simulink subsystem "DetailedBatteryModel"  (R2025b)
settings: Solver=VariableStepAuto  StartTime=0.0  StopTime=10.0  RelTol=1e-3
undefined symbols (not defined in the file): PlntBattBalSwtchThresh, PlntBattBleedRes, PlntBattCondArea, PlntBattNumCellPar, ThrmBatt1, ThrmBatt2, ThrmBatt3, ThrmBatt4
libraries: fl_lib x580, nesl_utility_internal x386, batteryecm_lib x96, simulink x96
(part 2 of 7)

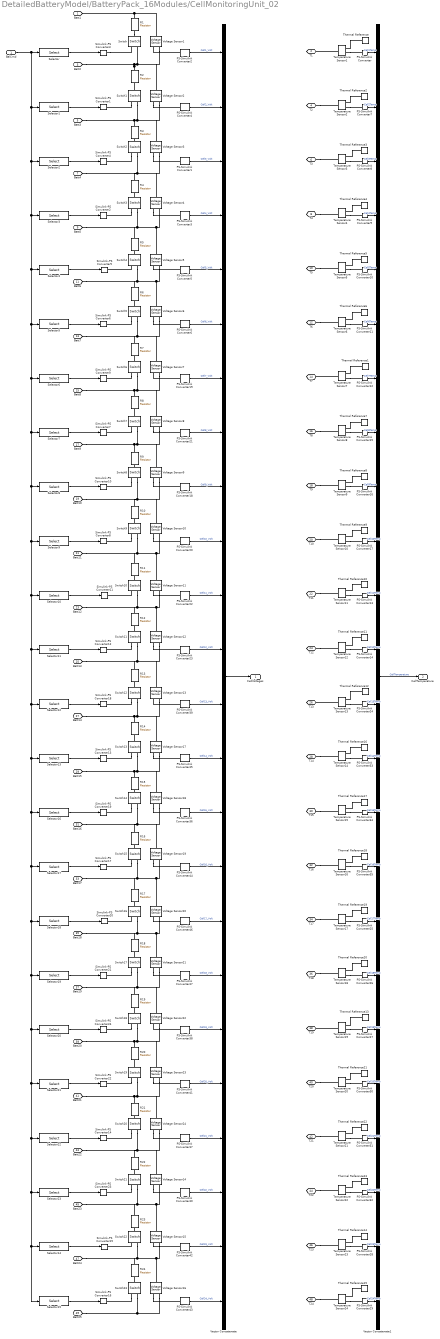
== system DetailedBatteryModel/BatteryPack_16Modules/CellMonitoringUnit_02 ==
  BalCmd : Inport
  PS-Simulink Converter{,7..17,24..35} (24 alike) : nesl_utility_internal/PS-Simulink Converter  PhysicalDomain=network_engine_domain  SubClassName=ps_output  LeftPortType=input  RightPortType=output  PseudoPeriodic=off  Frequencies=[]  VectorFormat=1-D array  Unit=degC  AffineConversion=on
  PS-Simulink Converter{1..6,18..23,36..47} (24 alike) : nesl_utility_internal/PS-Simulink Converter  PhysicalDomain=network_engine_domain  SubClassName=ps_output  LeftPortType=input  RightPortType=output  PseudoPeriodic=off  Frequencies=[]  VectorFormat=1-D array  Unit=V  AffineConversion=off
  R{1..24} (24 alike) : fl_lib/Electrical/Electrical Elements/Resistor  R=PlntBattBleedRes Ohm  i_specify=off  i_priority=None  i=0 A  i_nominal_specify=off  i_nominal_value=1  i_nominal_unit=A  v_specify=off  v_priority=None  v=0 V  v_nominal_specify=off  v_nominal_value=1  v_nominal_unit=V
      R1 settings: LogSimulationData=on
      R13 settings: LogSimulationData=on
      R19 settings: LogSimulationData=on
      R7 settings: LogSimulationData=on
  Selector : Selector  IndexOptions=Index vector (dialog)  Indices=1  OutputSizes=1
  Selector1 : Selector  IndexOptions=Index vector (dialog)  Indices=2  OutputSizes=1
  Selector10 : Selector  IndexOptions=Index vector (dialog)  Indices=11  OutputSizes=1
  Selector11 : Selector  IndexOptions=Index vector (dialog)  Indices=12  OutputSizes=1
  Selector12 : Selector  IndexOptions=Index vector (dialog)  Indices=13  OutputSizes=1
  Selector13 : Selector  IndexOptions=Index vector (dialog)  Indices=14  OutputSizes=1
  Selector14 : Selector  IndexOptions=Index vector (dialog)  Indices=23  OutputSizes=1
  Selector15 : Selector  IndexOptions=Index vector (dialog)  Indices=24  OutputSizes=1
  Selector16 : Selector  IndexOptions=Index vector (dialog)  Indices=15  OutputSizes=1
  Selector17 : Selector  IndexOptions=Index vector (dialog)  Indices=16  OutputSizes=1
  Selector18 : Selector  IndexOptions=Index vector (dialog)  Indices=17  OutputSizes=1
  Selector19 : Selector  IndexOptions=Index vector (dialog)  Indices=18  OutputSizes=1
  Selector2 : Selector  IndexOptions=Index vector (dialog)  Indices=3  OutputSizes=1
  Selector20 : Selector  IndexOptions=Index vector (dialog)  Indices=19  OutputSizes=1
  Selector21 : Selector  IndexOptions=Index vector (dialog)  Indices=20  OutputSizes=1
  Selector22 : Selector  IndexOptions=Index vector (dialog)  Indices=21  OutputSizes=1
  Selector23 : Selector  IndexOptions=Index vector (dialog)  Indices=22  OutputSizes=1
  Selector3 : Selector  IndexOptions=Index vector (dialog)  Indices=4  OutputSizes=1
  Selector4 : Selector  IndexOptions=Index vector (dialog)  Indices=5  OutputSizes=1
  Selector5 : Selector  IndexOptions=Index vector (dialog)  Indices=6  OutputSizes=1
  Selector6 : Selector  IndexOptions=Index vector (dialog)  Indices=7  OutputSizes=1
  Selector7 : Selector  IndexOptions=Index vector (dialog)  Indices=8  OutputSizes=1
  Selector8 : Selector  IndexOptions=Index vector (dialog)  Indices=9  OutputSizes=1
  Selector9 : Selector  IndexOptions=Index vector (dialog)  Indices=10  OutputSizes=1
  Simulink-PS Converter{1..24} (24 alike) : nesl_utility_internal/Simulink-PS Converter  PhysicalDomain=network_engine_domain  SubClassName=ps_input  LeftPortType=input  RightPortType=output  PseudoPeriodic=off  Frequencies=[]  NoiseDistribution=none  NoiseParameters=[]  Unit=1  AffineConversion=off  FilteringAndDerivatives=zero  SimscapeFilterOrder=1  InputFilterTimeConstant=0.001  UdotUserProvided=1
  Switch{,1..23} (24 alike) : fl_lib/Electrical/Electrical Elements/Switch  R_closed=PlntBattBalSwtchClsdRes Ohm  G_open=PlntBattBalSwtchOpenCond 1/Ohm  Threshold=PlntBattBalSwtchThresh  i_specify=off  i_priority=None  i=0 A  i_nominal_specify=off  i_nominal_value=1  i_nominal_unit=A  v_specify=off  v_priority=None  v=0 V  v_nominal_specify=off  v_nominal_value=1  v_nominal_unit=V
  Temperature Sensor{1..24} (24 alike) : fl_lib/Thermal/Thermal Sensors/Temperature Sensor  temperature_measure=foundation.enum.MeasurementReference.difference
  Thermal Reference{,1..23} (24 alike) : fl_lib/Thermal/Thermal Elements/Thermal Reference
  Vector Concatenate : Concatenate  NumInputs=24
  Vector Concatenate1 : Concatenate  NumInputs=24
  Voltage Sensor{1..24} (24 alike) : fl_lib/Electrical/Electrical Sensors/Voltage Sensor
  Batt1 : PMIOPort  Side=Left
  T1 : PMIOPort  Port=2  Side=Left
  Batt2 : PMIOPort  Port=3  Side=Left
  T2 : PMIOPort  Port=4  Side=Left
  Batt3 : PMIOPort  Port=5  Side=Left
  T3 : PMIOPort  Port=6  Side=Left
  Batt4 : PMIOPort  Port=7  Side=Left
  T4 : PMIOPort  Port=8  Side=Left
  Batt5 : PMIOPort  Port=9  Side=Left
  T5 : PMIOPort  Port=10  Side=Left
  Batt6 : PMIOPort  Port=11  Side=Left
  T6 : PMIOPort  Port=12  Side=Left
  Batt7 : PMIOPort  Port=13  Side=Left
  T7 : PMIOPort  Port=14  Side=Left
  Batt8 : PMIOPort  Port=15  Side=Left
  T8 : PMIOPort  Port=16  Side=Left
  Batt9 : PMIOPort  Port=17  Side=Left
  T9 : PMIOPort  Port=18  Side=Left
  Batt10 : PMIOPort  Port=19  Side=Left
  T10 : PMIOPort  Port=20  Side=Left
  Batt11 : PMIOPort  Port=21  Side=Left
  T11 : PMIOPort  Port=22  Side=Left
  Batt12 : PMIOPort  Port=23  Side=Left
  T12 : PMIOPort  Port=24  Side=Left
  Batt13 : PMIOPort  Port=25  Side=Left
  T13 : PMIOPort  Port=26  Side=Left
  Batt14 : PMIOPort  Port=27  Side=Left
  T14 : PMIOPort  Port=28  Side=Left
  Batt15 : PMIOPort  Port=29  Side=Left
  T15 : PMIOPort  Port=30  Side=Left
  Batt16 : PMIOPort  Port=31  Side=Left
  T16 : PMIOPort  Port=32  Side=Left
  Batt17 : PMIOPort  Port=33  Side=Left
  T17 : PMIOPort  Port=34  Side=Left
  Batt18 : PMIOPort  Port=35  Side=Left
  T18 : PMIOPort  Port=36  Side=Left
  Batt19 : PMIOPort  Port=37  Side=Left
  T19 : PMIOPort  Port=38  Side=Left
  Batt20 : PMIOPort  Port=39  Side=Left
  T20 : PMIOPort  Port=40  Side=Left
  Batt21 : PMIOPort  Port=41  Side=Left
  T21 : PMIOPort  Port=42  Side=Left
  Batt22 : PMIOPort  Port=43  Side=Left
  T22 : PMIOPort  Port=44  Side=Left
  Batt23 : PMIOPort  Port=45  Side=Left
  T23 : PMIOPort  Port=46  Side=Left
  Batt24 : PMIOPort  Port=47  Side=Left
  T24 : PMIOPort  Port=48  Side=Left
  Batt25 : PMIOPort  Port=49  Side=Left
  CellVoltages : Outport  VectorParamsAs1DForOutWhenUnconnected=off
  CellTemperature : Outport  Port=2  VectorParamsAs1DForOutWhenUnconnected=off
  wires:
  PS-Simulink Converter11/1 -> Vector Concatenate1/6  "Cell6Temp"
  PS-Simulink Converter10/1 -> Vector Concatenate1/5  "Cell5Temp"
  PS-Simulink Converter8/1 -> Vector Concatenate1/3  "Cell3Temp"
  PS-Simulink Converter7/1 -> Vector Concatenate1/2  "Cell2Temp"
  PS-Simulink Converter9/1 -> Vector Concatenate1/4  "Cell4Temp"
  PS-Simulink Converter/1 -> Vector Concatenate1/1  "Cell1Temp"
  Vector Concatenate1/1 -> CellTemperature/1  "CellTemperature"
  PS-Simulink Converter6/1 -> Vector Concatenate/6  "Cell6_Volt"
  PS-Simulink Converter5/1 -> Vector Concatenate/5  "Cell5_Volt"
  PS-Simulink Converter3/1 -> Vector Concatenate/4  "Cell4_Volt"
  PS-Simulink Converter1/1 -> Vector Concatenate/3  "Cell3_Volt"
  PS-Simulink Converter4/1 -> Vector Concatenate/2  "Cell2_Volt"
  PS-Simulink Converter2/1 -> Vector Concatenate/1  "Cell1_Volt"
  Selector5/1 -> Simulink-PS Converter6/1
  Selector4/1 -> Simulink-PS Converter5/1
  Selector3/1 -> Simulink-PS Converter2/1
  Selector/1 -> Simulink-PS Converter3/1
  Selector1/1 -> Simulink-PS Converter1/1
  Selector2/1 -> Simulink-PS Converter4/1
  Vector Concatenate/1 -> CellVoltages/1
  PS-Simulink Converter12/1 -> Vector Concatenate1/7  "Cell7Temp"
  PS-Simulink Converter15/1 -> Vector Concatenate1/8  "Cell8Temp"
  PS-Simulink Converter13/1 -> Vector Concatenate1/11  "Cell11Temp"
  PS-Simulink Converter17/1 -> Vector Concatenate1/10  "Cell10Temp"
  PS-Simulink Converter16/1 -> Vector Concatenate1/9  "Cell9Temp"
  PS-Simulink Converter14/1 -> Vector Concatenate1/12  "Cell12Temp"
  PS-Simulink Converter20/1 -> Vector Concatenate/10  "Cell10_Volt"
  Selector9/1 -> Simulink-PS Converter8/1
  Selector11/1 -> Simulink-PS Converter12/1
  Selector6/1 -> Simulink-PS Converter9/1
  PS-Simulink Converter18/1 -> Vector Concatenate/9  "Cell9_Volt"
  Selector8/1 -> Simulink-PS Converter10/1
  Selector7/1 -> Simulink-PS Converter7/1
  PS-Simulink Converter22/1 -> Vector Concatenate/11  "Cell11_Volt"
  PS-Simulink Converter23/1 -> Vector Concatenate/12  "Cell12_Volt"
  PS-Simulink Converter19/1 -> Vector Concatenate/7  "Cell7_Volt"
  PS-Simulink Converter21/1 -> Vector Concatenate/8  "Cell8_Volt"
  Selector10/1 -> Simulink-PS Converter11/1
  PS-Simulink Converter24/1 -> Vector Concatenate1/13  "Cell13Temp"
  PS-Simulink Converter33/1 -> Vector Concatenate1/14  "Cell14Temp"
  PS-Simulink Converter25/1 -> Vector Concatenate1/17  "Cell17Temp"
  PS-Simulink Converter30/1 -> Vector Concatenate1/20  "Cell20Temp"
  PS-Simulink Converter31/1 -> Vector Concatenate1/21  "Cell21Temp"
  PS-Simulink Converter28/1 -> Vector Concatenate1/23  "Cell23Temp"
  PS-Simulink Converter29/1 -> Vector Concatenate1/24  "Cell24Temp"
  PS-Simulink Converter27/1 -> Vector Concatenate1/19  "Cell19Temp"
  PS-Simulink Converter26/1 -> Vector Concatenate1/18  "Cell18Temp"
  PS-Simulink Converter34/1 -> Vector Concatenate1/15  "Cell15Temp"
  PS-Simulink Converter35/1 -> Vector Concatenate1/16  "Cell16Temp"
  PS-Simulink Converter32/1 -> Vector Concatenate1/22  "Cell22Temp"
  PS-Simulink Converter44/1 -> Vector Concatenate/16  "Cell16_Volt"
  Selector17/1 -> Simulink-PS Converter17/1
  Selector19/1 -> Simulink-PS Converter21/1
  Selector12/1 -> Simulink-PS Converter18/1
  PS-Simulink Converter36/1 -> Vector Concatenate/15  "Cell15_Volt"
  Selector13/1 -> Simulink-PS Converter13/1
  BalCmd/1 -> Selector/1, Selector1/1, Selector2/1, Selector4/1, Selector6/1, Selector7/1, Selector8/1, Selector10/1, Selector13/1, Selector16/1, Selector18/1, Selector20/1, Selector21/1, Selector22/1, Selector14/1, Selector15/1, Selector23/1, Selector19/1, Selector17/1, Selector12/1, Selector11/1, Selector9/1, Selector5/1, Selector3/1
  PS-Simulink Converter37/1 -> Vector Concatenate/21  "Cell21_Volt"
  PS-Simulink Converter38/1 -> Vector Concatenate/19  "Cell19_Volt"
  PS-Simulink Converter41/1 -> Vector Concatenate/20  "Cell20_Volt"
  PS-Simulink Converter43/1 -> Vector Concatenate/24  "Cell24_Volt"
  Selector15/1 -> Simulink-PS Converter16/1
  Selector20/1 -> Simulink-PS Converter24/1
  Selector22/1 -> Simulink-PS Converter14/1
  Selector14/1 -> Simulink-PS Converter15/1
  Selector21/1 -> Simulink-PS Converter22/1
  PS-Simulink Converter42/1 -> Vector Concatenate/23  "Cell23_Volt"
  Selector16/1 -> Simulink-PS Converter19/1
  PS-Simulink Converter46/1 -> Vector Concatenate/17  "Cell17_Volt"
  PS-Simulink Converter40/1 -> Vector Concatenate/22  "Cell22_Volt"
  PS-Simulink Converter47/1 -> Vector Concatenate/18  "Cell18_Volt"
  Selector23/1 -> Simulink-PS Converter23/1
  PS-Simulink Converter45/1 -> Vector Concatenate/14  "Cell14_Volt"
  Selector18/1 -> Simulink-PS Converter20/1
  PS-Simulink Converter39/1 -> Vector Concatenate/13  "Cell13_Volt"
  connections:
  Thermal Reference/LConn1 -- Temperature Sensor1/RConn1
  T6/RConn1 -- Temperature Sensor6/LConn1
  T5/RConn1 -- Temperature Sensor5/LConn1
  T4/RConn1 -- Temperature Sensor4/LConn1
  T3/RConn1 -- Temperature Sensor3/LConn1
  T2/RConn1 -- Temperature Sensor2/LConn1
  Temperature Sensor1/LConn1 -- T1/RConn1
  Thermal Reference5/LConn1 -- Temperature Sensor5/RConn1
  Thermal Reference2/LConn1 -- Temperature Sensor2/RConn1
  Thermal Reference6/LConn1 -- Temperature Sensor6/RConn1
  Temperature Sensor2/RConn2 -- PS-Simulink Converter7/LConn1
  Thermal Reference4/LConn1 -- Temperature Sensor4/RConn1
  Temperature Sensor5/RConn2 -- PS-Simulink Converter10/LConn1
  Thermal Reference3/LConn1 -- Temperature Sensor3/RConn1
  Temperature Sensor4/RConn2 -- PS-Simulink Converter9/LConn1
  Temperature Sensor6/RConn2 -- PS-Simulink Converter11/LConn1
  Temperature Sensor1/RConn2 -- PS-Simulink Converter/LConn1
  Temperature Sensor3/RConn2 -- PS-Simulink Converter8/LConn1
  Voltage Sensor6/RConn1 -- PS-Simulink Converter6/LConn1
  Voltage Sensor5/RConn1 -- PS-Simulink Converter5/LConn1
  Voltage Sensor4/RConn1 -- PS-Simulink Converter3/LConn1
  Switch5/LConn1 -- R6/RConn1
  Switch5/RConn1 -- Simulink-PS Converter6/RConn1
  Switch5/RConn2 -- R7/LConn1 -- Batt7/RConn1 -- Voltage Sensor6/RConn2 -- Voltage Sensor7/LConn1
  Switch4/LConn1 -- R5/RConn1
  Switch4/RConn1 -- Simulink-PS Converter5/RConn1
  Switch4/RConn2 -- Voltage Sensor5/RConn2 -- Voltage Sensor6/LConn1 -- R6/LConn1 -- Batt6/RConn1
  Switch3/RConn1 -- Simulink-PS Converter2/RConn1
  Switch3/LConn1 -- R4/RConn1
  Switch3/RConn2 -- Batt5/RConn1 -- R5/LConn1 -- Voltage Sensor5/LConn1 -- Voltage Sensor4/RConn2
  Switch1/RConn2 -- R3/LConn1 -- Batt3/RConn1 -- Voltage Sensor2/RConn2 -- Voltage Sensor3/LConn1
  R2/LConn1 -- Switch/RConn2 -- Voltage Sensor1/RConn2 -- Voltage Sensor2/LConn1 -- Batt2/RConn1
  R1/RConn1 -- Switch/LConn1
  Switch2/LConn1 -- R3/RConn1
  R1/LConn1 -- Voltage Sensor1/LConn1 -- Batt1/RConn1
  PS-Simulink Converter2/LConn1 -- Voltage Sensor1/RConn1
  Voltage Sensor2/RConn1 -- PS-Simulink Converter4/LConn1
  Switch1/LConn1 -- R2/RConn1
  Simulink-PS Converter3/RConn1 -- Switch/RConn1
  Switch1/RConn1 -- Simulink-PS Converter1/RConn1
  Switch2/RConn1 -- Simulink-PS Converter4/RConn1
  Voltage Sensor3/RConn1 -- PS-Simulink Converter1/LConn1
  Switch2/RConn2 -- R4/LConn1 -- Batt4/RConn1 -- Voltage Sensor3/RConn2 -- Voltage Sensor4/LConn1
  Temperature Sensor8/RConn2 -- PS-Simulink Converter15/LConn1
  Temperature Sensor11/RConn2 -- PS-Simulink Converter13/LConn1
  Thermal Reference9/LConn1 -- Temperature Sensor10/RConn1
  Temperature Sensor9/RConn2 -- PS-Simulink Converter16/LConn1
  Temperature Sensor10/RConn2 -- PS-Simulink Converter17/LConn1
  Thermal Reference11/LConn1 -- Temperature Sensor12/RConn1
  T10/RConn1 -- Temperature Sensor10/LConn1
  Thermal Reference10/LConn1 -- Temperature Sensor11/RConn1
  Temperature Sensor12/RConn2 -- PS-Simulink Converter14/LConn1
  Thermal Reference1/LConn1 -- Temperature Sensor7/RConn1
  T8/RConn1 -- Temperature Sensor8/LConn1
  Temperature Sensor7/LConn1 -- T7/RConn1
  T9/RConn1 -- Temperature Sensor9/LConn1
  T11/RConn1 -- Temperature Sensor11/LConn1
  Thermal Reference7/LConn1 -- Temperature Sensor8/RConn1
  T12/RConn1 -- Temperature Sensor12/LConn1
  Temperature Sensor7/RConn2 -- PS-Simulink Converter12/LConn1
  Thermal Reference8/LConn1 -- Temperature Sensor9/RConn1
  Switch8/RConn2 -- Voltage Sensor9/RConn2 -- Voltage Sensor10/LConn1 -- R10/LConn1 -- Batt10/RConn1
  Switch6/RConn2 -- R8/LConn1 -- Batt8/RConn1 -- Voltage Sensor7/RConn2 -- Voltage Sensor8/LConn1
  Switch10/RConn2 -- R12/LConn1 -- Batt12/RConn1 -- Voltage Sensor12/LConn1 -- Voltage Sensor11/RConn2
  Switch9/RConn2 -- Voltage Sensor10/RConn2 -- Voltage Sensor11/LConn1 -- R11/LConn1 -- Batt11/RConn1
  Switch7/RConn2 -- Voltage Sensor9/LConn1 -- Voltage Sensor8/RConn2 -- Batt9/RConn1 -- R9/LConn1
  Switch11/RConn2 -- R13/LConn1 -- Batt13/RConn1 -- Voltage Sensor12/RConn2 -- Voltage Sensor13/LConn1
  Switch9/LConn1 -- R10/RConn1
  Switch7/RConn1 -- Simulink-PS Converter7/RConn1
  Switch6/LConn1 -- R7/RConn1
  Voltage Sensor12/RConn1 -- PS-Simulink Converter23/LConn1
  Voltage Sensor10/RConn1 -- PS-Simulink Converter20/LConn1
  Switch7/LConn1 -- R8/RConn1
  Voltage Sensor8/RConn1 -- PS-Simulink Converter21/LConn1
  Voltage Sensor9/RConn1 -- PS-Simulink Converter18/LConn1
  Switch6/RConn1 -- Simulink-PS Converter9/RConn1
  PS-Simulink Converter19/LConn1 -- Voltage Sensor7/RConn1
  Switch8/LConn1 -- R9/RConn1
  Voltage Sensor11/RConn1 -- PS-Simulink Converter22/LConn1
  Switch9/RConn1 -- Simulink-PS Converter8/RConn1
  Switch10/RConn1 -- Simulink-PS Converter11/RConn1
  Switch10/LConn1 -- R11/RConn1
  Switch11/RConn1 -- Simulink-PS Converter12/RConn1
  Switch11/LConn1 -- R12/RConn1
  Switch8/RConn1 -- Simulink-PS Converter10/RConn1
  Thermal Reference20/LConn1 -- Temperature Sensor18/RConn1
  T16/RConn1 -- Temperature Sensor16/LConn1
  Thermal Reference18/LConn1 -- Temperature Sensor16/RConn1
  Thermal Reference19/LConn1 -- Temperature Sensor17/RConn1
  T17/RConn1 -- Temperature Sensor17/LConn1
  Temperature Sensor13/LConn1 -- T13/RConn1
  Temperature Sensor17/RConn2 -- PS-Simulink Converter25/LConn1
  Temperature Sensor16/RConn2 -- PS-Simulink Converter35/LConn1
  Thermal Reference16/LConn1 -- Temperature Sensor14/RConn1
  T20/RConn1 -- Temperature Sensor20/LConn1
  Temperature Sensor15/RConn2 -- PS-Simulink Converter34/LConn1
  Thermal Reference17/LConn1 -- Temperature Sensor15/RConn1
  Temperature Sensor21/RConn2 -- PS-Simulink Converter31/LConn1
  Thermal Reference13/LConn1 -- Temperature Sensor19/RConn1
  Thermal Reference14/LConn1 -- Temperature Sensor23/RConn1
  Thermal Reference15/LConn1 -- Temperature Sensor24/RConn1
  Thermal Reference12/LConn1 -- Temperature Sensor13/RConn1
  Temperature Sensor18/RConn2 -- PS-Simulink Converter26/LConn1
  T14/RConn1 -- Temperature Sensor14/LConn1
  T22/RConn1 -- Temperature Sensor22/LConn1
  Thermal Reference23/LConn1 -- Temperature Sensor22/RConn1
  Temperature Sensor13/RConn2 -- PS-Simulink Converter24/LConn1
  Temperature Sensor24/RConn2 -- PS-Simulink Converter29/LConn1
  Thermal Reference22/LConn1 -- Temperature Sensor21/RConn1
  T21/RConn1 -- Temperature Sensor21/LConn1
  T18/RConn1 -- Temperature Sensor18/LConn1
  T15/RConn1 -- Temperature Sensor15/LConn1
  T23/RConn1 -- Temperature Sensor23/LConn1
  T24/RConn1 -- Temperature Sensor24/LConn1
  Temperature Sensor19/LConn1 -- T19/RConn1
  Temperature Sensor23/RConn2 -- PS-Simulink Converter28/LConn1
  Temperature Sensor19/RConn2 -- PS-Simulink Converter27/LConn1
  Temperature Sensor14/RConn2 -- PS-Simulink Converter33/LConn1
  Thermal Reference21/LConn1 -- Temperature Sensor20/RConn1
  Temperature Sensor20/RConn2 -- PS-Simulink Converter30/LConn1
  Temperature Sensor22/RConn2 -- PS-Simulink Converter32/LConn1
  Switch20/RConn2 -- Voltage Sensor24/RConn2 -- Voltage Sensor14/LConn1 -- R22/LConn1 -- Batt22/RConn1
  Switch16/RConn2 -- R18/LConn1 -- Batt18/RConn1 -- Voltage Sensor21/LConn1 -- Voltage Sensor20/RConn2
  Switch14/RConn2 -- R16/LConn1 -- Batt16/RConn1 -- Voltage Sensor19/LConn1 -- Voltage Sensor18/RConn2
  Switch22/RConn2 -- R24/LConn1 -- Batt24/RConn1 -- Voltage Sensor16/LConn1 -- Voltage Sensor15/RConn2
  Switch19/RConn2 -- Voltage Sensor24/LConn1 -- Voltage Sensor23/RConn2 -- Batt21/RConn1 -- R21/LConn1
  Switch21/RConn2 -- Voltage Sensor14/RConn2 -- Voltage Sensor15/LConn1 -- Batt23/RConn1 -- R23/LConn1
  Switch12/RConn2 -- R14/LConn1 -- Batt14/RConn1 -- Voltage Sensor13/RConn2 -- Voltage Sensor17/LConn1
  Switch15/RConn2 -- Voltage Sensor19/RConn2 -- Voltage Sensor20/LConn1 -- R17/LConn1 -- Batt17/RConn1
  Switch13/RConn2 -- R15/LConn1 -- Batt15/RConn1 -- Voltage Sensor18/LConn1 -- Voltage Sensor17/RConn2
  Switch17/RConn2 -- R19/LConn1 -- Batt19/RConn1 -- Voltage Sensor21/RConn2 -- Voltage Sensor22/LConn1
  Switch18/RConn2 -- Voltage Sensor22/RConn2 -- Voltage Sensor23/LConn1 -- Batt20/RConn1 -- R20/LConn1
  Switch23/RConn2 -- Batt25/RConn1 -- Voltage Sensor16/RConn2
  Switch14/RConn1 -- Simulink-PS Converter19/RConn1
  Switch22/RConn1 -- Simulink-PS Converter15/RConn1
  Voltage Sensor21/RConn1 -- PS-Simulink Converter47/LConn1
  Switch13/LConn1 -- R14/RConn1
  PS-Simulink Converter39/LConn1 -- Voltage Sensor13/RConn1
  Voltage Sensor19/RConn1 -- PS-Simulink Converter44/LConn1
  Switch21/RConn1 -- Simulink-PS Converter23/RConn1
  Voltage Sensor23/RConn1 -- PS-Simulink Converter41/LConn1
  Voltage Sensor18/RConn1 -- PS-Simulink Converter36/LConn1
  Voltage Sensor17/RConn1 -- PS-Simulink Converter45/LConn1
  Switch23/LConn1 -- R24/RConn1
  Switch12/LConn1 -- R13/RConn1
  PS-Simulink Converter38/LConn1 -- Voltage Sensor22/RConn1
  Switch18/RConn1 -- Simulink-PS Converter24/RConn1
  Switch12/RConn1 -- Simulink-PS Converter18/RConn1
  Switch13/RConn1 -- Simulink-PS Converter13/RConn1
  Switch15/LConn1 -- R16/RConn1
  Switch20/LConn1 -- R21/RConn1
  Switch14/LConn1 -- R15/RConn1
  Voltage Sensor14/RConn1 -- PS-Simulink Converter40/LConn1
  Voltage Sensor20/RConn1 -- PS-Simulink Converter46/LConn1
  Voltage Sensor16/RConn1 -- PS-Simulink Converter43/LConn1
  Switch18/LConn1 -- R19/RConn1
  Switch21/LConn1 -- R22/RConn1
  Switch17/LConn1 -- R18/RConn1
  Switch16/RConn1 -- Simulink-PS Converter20/RConn1
  Switch19/RConn1 -- Simulink-PS Converter22/RConn1
  Switch16/LConn1 -- R17/RConn1
  Voltage Sensor15/RConn1 -- PS-Simulink Converter42/LConn1
  Switch17/RConn1 -- Simulink-PS Converter21/RConn1
  Switch23/RConn1 -- Simulink-PS Converter16/RConn1
  Switch20/RConn1 -- Simulink-PS Converter14/RConn1
  Switch22/LConn1 -- R23/RConn1
  Switch19/LConn1 -- R20/RConn1
  Switch15/RConn1 -- Simulink-PS Converter17/RConn1
  Voltage Sensor24/RConn1 -- PS-Simulink Converter37/LConn1

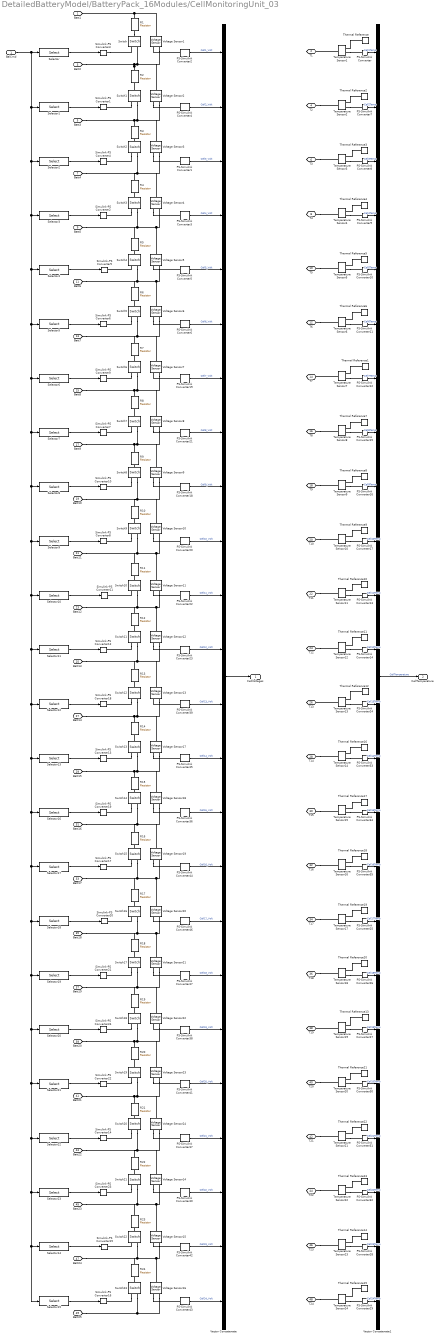
== system DetailedBatteryModel/BatteryPack_16Modules/CellMonitoringUnit_03 ==
  BalCmd : Inport
  PS-Simulink Converter{,7..17,24..35} (24 alike) : nesl_utility_internal/PS-Simulink Converter  PhysicalDomain=network_engine_domain  SubClassName=ps_output  LeftPortType=input  RightPortType=output  PseudoPeriodic=off  Frequencies=[]  VectorFormat=1-D array  Unit=degC  AffineConversion=on
  PS-Simulink Converter{1..6,18..23,36..47} (24 alike) : nesl_utility_internal/PS-Simulink Converter  PhysicalDomain=network_engine_domain  SubClassName=ps_output  LeftPortType=input  RightPortType=output  PseudoPeriodic=off  Frequencies=[]  VectorFormat=1-D array  Unit=V  AffineConversion=off
  R{1..24} (24 alike) : fl_lib/Electrical/Electrical Elements/Resistor  R=PlntBattBleedRes Ohm  i_specify=off  i_priority=None  i=0 A  i_nominal_specify=off  i_nominal_value=1  i_nominal_unit=A  v_specify=off  v_priority=None  v=0 V  v_nominal_specify=off  v_nominal_value=1  v_nominal_unit=V
      R1 settings: LogSimulationData=on
      R13 settings: LogSimulationData=on
      R19 settings: LogSimulationData=on
      R7 settings: LogSimulationData=on
  Selector : Selector  IndexOptions=Index vector (dialog)  Indices=1  OutputSizes=1
  Selector1 : Selector  IndexOptions=Index vector (dialog)  Indices=2  OutputSizes=1
  Selector10 : Selector  IndexOptions=Index vector (dialog)  Indices=11  OutputSizes=1
  Selector11 : Selector  IndexOptions=Index vector (dialog)  Indices=12  OutputSizes=1
  Selector12 : Selector  IndexOptions=Index vector (dialog)  Indices=13  OutputSizes=1
  Selector13 : Selector  IndexOptions=Index vector (dialog)  Indices=14  OutputSizes=1
  Selector14 : Selector  IndexOptions=Index vector (dialog)  Indices=23  OutputSizes=1
  Selector15 : Selector  IndexOptions=Index vector (dialog)  Indices=24  OutputSizes=1
  Selector16 : Selector  IndexOptions=Index vector (dialog)  Indices=15  OutputSizes=1
  Selector17 : Selector  IndexOptions=Index vector (dialog)  Indices=16  OutputSizes=1
  Selector18 : Selector  IndexOptions=Index vector (dialog)  Indices=17  OutputSizes=1
  Selector19 : Selector  IndexOptions=Index vector (dialog)  Indices=18  OutputSizes=1
  Selector2 : Selector  IndexOptions=Index vector (dialog)  Indices=3  OutputSizes=1
  Selector20 : Selector  IndexOptions=Index vector (dialog)  Indices=19  OutputSizes=1
  Selector21 : Selector  IndexOptions=Index vector (dialog)  Indices=20  OutputSizes=1
  Selector22 : Selector  IndexOptions=Index vector (dialog)  Indices=21  OutputSizes=1
  Selector23 : Selector  IndexOptions=Index vector (dialog)  Indices=22  OutputSizes=1
  Selector3 : Selector  IndexOptions=Index vector (dialog)  Indices=4  OutputSizes=1
  Selector4 : Selector  IndexOptions=Index vector (dialog)  Indices=5  OutputSizes=1
  Selector5 : Selector  IndexOptions=Index vector (dialog)  Indices=6  OutputSizes=1
  Selector6 : Selector  IndexOptions=Index vector (dialog)  Indices=7  OutputSizes=1
  Selector7 : Selector  IndexOptions=Index vector (dialog)  Indices=8  OutputSizes=1
  Selector8 : Selector  IndexOptions=Index vector (dialog)  Indices=9  OutputSizes=1
  Selector9 : Selector  IndexOptions=Index vector (dialog)  Indices=10  OutputSizes=1
  Simulink-PS Converter{1..24} (24 alike) : nesl_utility_internal/Simulink-PS Converter  PhysicalDomain=network_engine_domain  SubClassName=ps_input  LeftPortType=input  RightPortType=output  PseudoPeriodic=off  Frequencies=[]  NoiseDistribution=none  NoiseParameters=[]  Unit=1  AffineConversion=off  FilteringAndDerivatives=zero  SimscapeFilterOrder=1  InputFilterTimeConstant=0.001  UdotUserProvided=1
  Switch{,1..23} (24 alike) : fl_lib/Electrical/Electrical Elements/Switch  R_closed=PlntBattBalSwtchClsdRes Ohm  G_open=PlntBattBalSwtchOpenCond 1/Ohm  Threshold=PlntBattBalSwtchThresh  i_specify=off  i_priority=None  i=0 A  i_nominal_specify=off  i_nominal_value=1  i_nominal_unit=A  v_specify=off  v_priority=None  v=0 V  v_nominal_specify=off  v_nominal_value=1  v_nominal_unit=V
  Temperature Sensor{1..24} (24 alike) : fl_lib/Thermal/Thermal Sensors/Temperature Sensor  temperature_measure=foundation.enum.MeasurementReference.difference
  Thermal Reference{,1..23} (24 alike) : fl_lib/Thermal/Thermal Elements/Thermal Reference
  Vector Concatenate : Concatenate  NumInputs=24
  Vector Concatenate1 : Concatenate  NumInputs=24
  Voltage Sensor{1..24} (24 alike) : fl_lib/Electrical/Electrical Sensors/Voltage Sensor
  Batt1 : PMIOPort  Side=Left
  T1 : PMIOPort  Port=2  Side=Left
  Batt2 : PMIOPort  Port=3  Side=Left
  T2 : PMIOPort  Port=4  Side=Left
  Batt3 : PMIOPort  Port=5  Side=Left
  T3 : PMIOPort  Port=6  Side=Left
  Batt4 : PMIOPort  Port=7  Side=Left
  T4 : PMIOPort  Port=8  Side=Left
  Batt5 : PMIOPort  Port=9  Side=Left
  T5 : PMIOPort  Port=10  Side=Left
  Batt6 : PMIOPort  Port=11  Side=Left
  T6 : PMIOPort  Port=12  Side=Left
  Batt7 : PMIOPort  Port=13  Side=Left
  T7 : PMIOPort  Port=14  Side=Left
  Batt8 : PMIOPort  Port=15  Side=Left
  T8 : PMIOPort  Port=16  Side=Left
  Batt9 : PMIOPort  Port=17  Side=Left
  T9 : PMIOPort  Port=18  Side=Left
  Batt10 : PMIOPort  Port=19  Side=Left
  T10 : PMIOPort  Port=20  Side=Left
  Batt11 : PMIOPort  Port=21  Side=Left
  T11 : PMIOPort  Port=22  Side=Left
  Batt12 : PMIOPort  Port=23  Side=Left
  T12 : PMIOPort  Port=24  Side=Left
  Batt13 : PMIOPort  Port=25  Side=Left
  T13 : PMIOPort  Port=26  Side=Left
  Batt14 : PMIOPort  Port=27  Side=Left
  T14 : PMIOPort  Port=28  Side=Left
  Batt15 : PMIOPort  Port=29  Side=Left
  T15 : PMIOPort  Port=30  Side=Left
  Batt16 : PMIOPort  Port=31  Side=Left
  T16 : PMIOPort  Port=32  Side=Left
  Batt17 : PMIOPort  Port=33  Side=Left
  T17 : PMIOPort  Port=34  Side=Left
  Batt18 : PMIOPort  Port=35  Side=Left
  T18 : PMIOPort  Port=36  Side=Left
  Batt19 : PMIOPort  Port=37  Side=Left
  T19 : PMIOPort  Port=38  Side=Left
  Batt20 : PMIOPort  Port=39  Side=Left
  T20 : PMIOPort  Port=40  Side=Left
  Batt21 : PMIOPort  Port=41  Side=Left
  T21 : PMIOPort  Port=42  Side=Left
  Batt22 : PMIOPort  Port=43  Side=Left
  T22 : PMIOPort  Port=44  Side=Left
  Batt23 : PMIOPort  Port=45  Side=Left
  T23 : PMIOPort  Port=46  Side=Left
  Batt24 : PMIOPort  Port=47  Side=Left
  T24 : PMIOPort  Port=48  Side=Left
  Batt25 : PMIOPort  Port=49  Side=Left
  CellVoltages : Outport  VectorParamsAs1DForOutWhenUnconnected=off
  CellTemperature : Outport  Port=2  VectorParamsAs1DForOutWhenUnconnected=off
  wires:
  PS-Simulink Converter11/1 -> Vector Concatenate1/6  "Cell6Temp"
  PS-Simulink Converter10/1 -> Vector Concatenate1/5  "Cell5Temp"
  PS-Simulink Converter8/1 -> Vector Concatenate1/3  "Cell3Temp"
  PS-Simulink Converter7/1 -> Vector Concatenate1/2  "Cell2Temp"
  PS-Simulink Converter9/1 -> Vector Concatenate1/4  "Cell4Temp"
  PS-Simulink Converter/1 -> Vector Concatenate1/1  "Cell1Temp"
  Vector Concatenate1/1 -> CellTemperature/1  "CellTemperature"
  PS-Simulink Converter6/1 -> Vector Concatenate/6  "Cell6_Volt"
  PS-Simulink Converter5/1 -> Vector Concatenate/5  "Cell5_Volt"
  PS-Simulink Converter3/1 -> Vector Concatenate/4  "Cell4_Volt"
  PS-Simulink Converter1/1 -> Vector Concatenate/3  "Cell3_Volt"
  PS-Simulink Converter4/1 -> Vector Concatenate/2  "Cell2_Volt"
  PS-Simulink Converter2/1 -> Vector Concatenate/1  "Cell1_Volt"
  Selector5/1 -> Simulink-PS Converter6/1
  Selector4/1 -> Simulink-PS Converter5/1
  Selector3/1 -> Simulink-PS Converter2/1
  Selector/1 -> Simulink-PS Converter3/1
  Selector1/1 -> Simulink-PS Converter1/1
  Selector2/1 -> Simulink-PS Converter4/1
  Vector Concatenate/1 -> CellVoltages/1
  PS-Simulink Converter12/1 -> Vector Concatenate1/7  "Cell7Temp"
  PS-Simulink Converter15/1 -> Vector Concatenate1/8  "Cell8Temp"
  PS-Simulink Converter13/1 -> Vector Concatenate1/11  "Cell11Temp"
  PS-Simulink Converter17/1 -> Vector Concatenate1/10  "Cell10Temp"
  PS-Simulink Converter16/1 -> Vector Concatenate1/9  "Cell9Temp"
  PS-Simulink Converter14/1 -> Vector Concatenate1/12  "Cell12Temp"
  PS-Simulink Converter20/1 -> Vector Concatenate/10  "Cell10_Volt"
  Selector9/1 -> Simulink-PS Converter8/1
  Selector11/1 -> Simulink-PS Converter12/1
  Selector6/1 -> Simulink-PS Converter9/1
  PS-Simulink Converter18/1 -> Vector Concatenate/9  "Cell9_Volt"
  Selector8/1 -> Simulink-PS Converter10/1
  Selector7/1 -> Simulink-PS Converter7/1
  PS-Simulink Converter22/1 -> Vector Concatenate/11  "Cell11_Volt"
  PS-Simulink Converter23/1 -> Vector Concatenate/12  "Cell12_Volt"
  PS-Simulink Converter19/1 -> Vector Concatenate/7  "Cell7_Volt"
  PS-Simulink Converter21/1 -> Vector Concatenate/8  "Cell8_Volt"
  Selector10/1 -> Simulink-PS Converter11/1
  PS-Simulink Converter24/1 -> Vector Concatenate1/13  "Cell13Temp"
  PS-Simulink Converter33/1 -> Vector Concatenate1/14  "Cell14Temp"
  PS-Simulink Converter25/1 -> Vector Concatenate1/17  "Cell17Temp"
  PS-Simulink Converter30/1 -> Vector Concatenate1/20  "Cell20Temp"
  PS-Simulink Converter31/1 -> Vector Concatenate1/21  "Cell21Temp"
  PS-Simulink Converter28/1 -> Vector Concatenate1/23  "Cell23Temp"
  PS-Simulink Converter29/1 -> Vector Concatenate1/24  "Cell24Temp"
  PS-Simulink Converter27/1 -> Vector Concatenate1/19  "Cell19Temp"
  PS-Simulink Converter26/1 -> Vector Concatenate1/18  "Cell18Temp"
  PS-Simulink Converter34/1 -> Vector Concatenate1/15  "Cell15Temp"
  PS-Simulink Converter35/1 -> Vector Concatenate1/16  "Cell16Temp"
  PS-Simulink Converter32/1 -> Vector Concatenate1/22  "Cell22Temp"
  PS-Simulink Converter44/1 -> Vector Concatenate/16  "Cell16_Volt"
  Selector17/1 -> Simulink-PS Converter17/1
  Selector19/1 -> Simulink-PS Converter21/1
  Selector12/1 -> Simulink-PS Converter18/1
  PS-Simulink Converter36/1 -> Vector Concatenate/15  "Cell15_Volt"
  Selector13/1 -> Simulink-PS Converter13/1
  BalCmd/1 -> Selector/1, Selector1/1, Selector2/1, Selector4/1, Selector6/1, Selector7/1, Selector8/1, Selector10/1, Selector13/1, Selector16/1, Selector18/1, Selector20/1, Selector21/1, Selector22/1, Selector14/1, Selector15/1, Selector23/1, Selector19/1, Selector17/1, Selector12/1, Selector11/1, Selector9/1, Selector5/1, Selector3/1
  PS-Simulink Converter37/1 -> Vector Concatenate/21  "Cell21_Volt"
  PS-Simulink Converter38/1 -> Vector Concatenate/19  "Cell19_Volt"
  PS-Simulink Converter41/1 -> Vector Concatenate/20  "Cell20_Volt"
  PS-Simulink Converter43/1 -> Vector Concatenate/24  "Cell24_Volt"
  Selector15/1 -> Simulink-PS Converter16/1
  Selector20/1 -> Simulink-PS Converter24/1
  Selector22/1 -> Simulink-PS Converter14/1
  Selector14/1 -> Simulink-PS Converter15/1
  Selector21/1 -> Simulink-PS Converter22/1
  PS-Simulink Converter42/1 -> Vector Concatenate/23  "Cell23_Volt"
  Selector16/1 -> Simulink-PS Converter19/1
  PS-Simulink Converter46/1 -> Vector Concatenate/17  "Cell17_Volt"
  PS-Simulink Converter40/1 -> Vector Concatenate/22  "Cell22_Volt"
  PS-Simulink Converter47/1 -> Vector Concatenate/18  "Cell18_Volt"
  Selector23/1 -> Simulink-PS Converter23/1
  PS-Simulink Converter45/1 -> Vector Concatenate/14  "Cell14_Volt"
  Selector18/1 -> Simulink-PS Converter20/1
  PS-Simulink Converter39/1 -> Vector Concatenate/13  "Cell13_Volt"
  connections:
  Thermal Reference/LConn1 -- Temperature Sensor1/RConn1
  T6/RConn1 -- Temperature Sensor6/LConn1
  T5/RConn1 -- Temperature Sensor5/LConn1
  T4/RConn1 -- Temperature Sensor4/LConn1
  T3/RConn1 -- Temperature Sensor3/LConn1
  T2/RConn1 -- Temperature Sensor2/LConn1
  Temperature Sensor1/LConn1 -- T1/RConn1
  Thermal Reference5/LConn1 -- Temperature Sensor5/RConn1
  Thermal Reference2/LConn1 -- Temperature Sensor2/RConn1
  Thermal Reference6/LConn1 -- Temperature Sensor6/RConn1
  Temperature Sensor2/RConn2 -- PS-Simulink Converter7/LConn1
  Thermal Reference4/LConn1 -- Temperature Sensor4/RConn1
  Temperature Sensor5/RConn2 -- PS-Simulink Converter10/LConn1
  Thermal Reference3/LConn1 -- Temperature Sensor3/RConn1
  Temperature Sensor4/RConn2 -- PS-Simulink Converter9/LConn1
  Temperature Sensor6/RConn2 -- PS-Simulink Converter11/LConn1
  Temperature Sensor1/RConn2 -- PS-Simulink Converter/LConn1
  Temperature Sensor3/RConn2 -- PS-Simulink Converter8/LConn1
  Voltage Sensor6/RConn1 -- PS-Simulink Converter6/LConn1
  Voltage Sensor5/RConn1 -- PS-Simulink Converter5/LConn1
  Voltage Sensor4/RConn1 -- PS-Simulink Converter3/LConn1
  Switch5/LConn1 -- R6/RConn1
  Switch5/RConn1 -- Simulink-PS Converter6/RConn1
  Switch5/RConn2 -- R7/LConn1 -- Batt7/RConn1 -- Voltage Sensor6/RConn2 -- Voltage Sensor7/LConn1
  Switch4/LConn1 -- R5/RConn1
  Switch4/RConn1 -- Simulink-PS Converter5/RConn1
  Switch4/RConn2 -- Voltage Sensor5/RConn2 -- Voltage Sensor6/LConn1 -- R6/LConn1 -- Batt6/RConn1
  Switch3/RConn1 -- Simulink-PS Converter2/RConn1
  Switch3/LConn1 -- R4/RConn1
  Switch3/RConn2 -- Batt5/RConn1 -- R5/LConn1 -- Voltage Sensor5/LConn1 -- Voltage Sensor4/RConn2
  Switch1/RConn2 -- R3/LConn1 -- Batt3/RConn1 -- Voltage Sensor2/RConn2 -- Voltage Sensor3/LConn1
  R2/LConn1 -- Switch/RConn2 -- Voltage Sensor1/RConn2 -- Voltage Sensor2/LConn1 -- Batt2/RConn1
  R1/RConn1 -- Switch/LConn1
  Switch2/LConn1 -- R3/RConn1
  R1/LConn1 -- Voltage Sensor1/LConn1 -- Batt1/RConn1
  PS-Simulink Converter2/LConn1 -- Voltage Sensor1/RConn1
  Voltage Sensor2/RConn1 -- PS-Simulink Converter4/LConn1
  Switch1/LConn1 -- R2/RConn1
  Simulink-PS Converter3/RConn1 -- Switch/RConn1
  Switch1/RConn1 -- Simulink-PS Converter1/RConn1
  Switch2/RConn1 -- Simulink-PS Converter4/RConn1
  Voltage Sensor3/RConn1 -- PS-Simulink Converter1/LConn1
  Switch2/RConn2 -- R4/LConn1 -- Batt4/RConn1 -- Voltage Sensor3/RConn2 -- Voltage Sensor4/LConn1
  Temperature Sensor8/RConn2 -- PS-Simulink Converter15/LConn1
  Temperature Sensor11/RConn2 -- PS-Simulink Converter13/LConn1
  Thermal Reference9/LConn1 -- Temperature Sensor10/RConn1
  Temperature Sensor9/RConn2 -- PS-Simulink Converter16/LConn1
  Temperature Sensor10/RConn2 -- PS-Simulink Converter17/LConn1
  Thermal Reference11/LConn1 -- Temperature Sensor12/RConn1
  T10/RConn1 -- Temperature Sensor10/LConn1
  Thermal Reference10/LConn1 -- Temperature Sensor11/RConn1
  Temperature Sensor12/RConn2 -- PS-Simulink Converter14/LConn1
  Thermal Reference1/LConn1 -- Temperature Sensor7/RConn1
  T8/RConn1 -- Temperature Sensor8/LConn1
  Temperature Sensor7/LConn1 -- T7/RConn1
  T9/RConn1 -- Temperature Sensor9/LConn1
  T11/RConn1 -- Temperature Sensor11/LConn1
  Thermal Reference7/LConn1 -- Temperature Sensor8/RConn1
  T12/RConn1 -- Temperature Sensor12/LConn1
  Temperature Sensor7/RConn2 -- PS-Simulink Converter12/LConn1
  Thermal Reference8/LConn1 -- Temperature Sensor9/RConn1
  Switch8/RConn2 -- Voltage Sensor9/RConn2 -- Voltage Sensor10/LConn1 -- R10/LConn1 -- Batt10/RConn1
  Switch6/RConn2 -- R8/LConn1 -- Batt8/RConn1 -- Voltage Sensor7/RConn2 -- Voltage Sensor8/LConn1
  Switch10/RConn2 -- R12/LConn1 -- Batt12/RConn1 -- Voltage Sensor12/LConn1 -- Voltage Sensor11/RConn2
  Switch9/RConn2 -- Voltage Sensor10/RConn2 -- Voltage Sensor11/LConn1 -- R11/LConn1 -- Batt11/RConn1
  Switch7/RConn2 -- Voltage Sensor9/LConn1 -- Voltage Sensor8/RConn2 -- Batt9/RConn1 -- R9/LConn1
  Switch11/RConn2 -- R13/LConn1 -- Batt13/RConn1 -- Voltage Sensor12/RConn2 -- Voltage Sensor13/LConn1
  Switch9/LConn1 -- R10/RConn1
  Switch7/RConn1 -- Simulink-PS Converter7/RConn1
  Switch6/LConn1 -- R7/RConn1
  Voltage Sensor12/RConn1 -- PS-Simulink Converter23/LConn1
  Voltage Sensor10/RConn1 -- PS-Simulink Converter20/LConn1
  Switch7/LConn1 -- R8/RConn1
  Voltage Sensor8/RConn1 -- PS-Simulink Converter21/LConn1
  Voltage Sensor9/RConn1 -- PS-Simulink Converter18/LConn1
  Switch6/RConn1 -- Simulink-PS Converter9/RConn1
  PS-Simulink Converter19/LConn1 -- Voltage Sensor7/RConn1
  Switch8/LConn1 -- R9/RConn1
  Voltage Sensor11/RConn1 -- PS-Simulink Converter22/LConn1
  Switch9/RConn1 -- Simulink-PS Converter8/RConn1
  Switch10/RConn1 -- Simulink-PS Converter11/RConn1
  Switch10/LConn1 -- R11/RConn1
  Switch11/RConn1 -- Simulink-PS Converter12/RConn1
  Switch11/LConn1 -- R12/RConn1
  Switch8/RConn1 -- Simulink-PS Converter10/RConn1
  Thermal Reference20/LConn1 -- Temperature Sensor18/RConn1
  T16/RConn1 -- Temperature Sensor16/LConn1
  Thermal Reference18/LConn1 -- Temperature Sensor16/RConn1
  Thermal Reference19/LConn1 -- Temperature Sensor17/RConn1
  T17/RConn1 -- Temperature Sensor17/LConn1
  Temperature Sensor13/LConn1 -- T13/RConn1
  Temperature Sensor17/RConn2 -- PS-Simulink Converter25/LConn1
  Temperature Sensor16/RConn2 -- PS-Simulink Converter35/LConn1
  Thermal Reference16/LConn1 -- Temperature Sensor14/RConn1
  T20/RConn1 -- Temperature Sensor20/LConn1
  Temperature Sensor15/RConn2 -- PS-Simulink Converter34/LConn1
  Thermal Reference17/LConn1 -- Temperature Sensor15/RConn1
  Temperature Sensor21/RConn2 -- PS-Simulink Converter31/LConn1
  Thermal Reference13/LConn1 -- Temperature Sensor19/RConn1
  Thermal Reference14/LConn1 -- Temperature Sensor23/RConn1
  Thermal Reference15/LConn1 -- Temperature Sensor24/RConn1
  Thermal Reference12/LConn1 -- Temperature Sensor13/RConn1
  Temperature Sensor18/RConn2 -- PS-Simulink Converter26/LConn1
  T14/RConn1 -- Temperature Sensor14/LConn1
  T22/RConn1 -- Temperature Sensor22/LConn1
  Thermal Reference23/LConn1 -- Temperature Sensor22/RConn1
  Temperature Sensor13/RConn2 -- PS-Simulink Converter24/LConn1
  Temperature Sensor24/RConn2 -- PS-Simulink Converter29/LConn1
  Thermal Reference22/LConn1 -- Temperature Sensor21/RConn1
  T21/RConn1 -- Temperature Sensor21/LConn1
  T18/RConn1 -- Temperature Sensor18/LConn1
  T15/RConn1 -- Temperature Sensor15/LConn1
  T23/RConn1 -- Temperature Sensor23/LConn1
  T24/RConn1 -- Temperature Sensor24/LConn1
  Temperature Sensor19/LConn1 -- T19/RConn1
  Temperature Sensor23/RConn2 -- PS-Simulink Converter28/LConn1
  Temperature Sensor19/RConn2 -- PS-Simulink Converter27/LConn1
  Temperature Sensor14/RConn2 -- PS-Simulink Converter33/LConn1
  Thermal Reference21/LConn1 -- Temperature Sensor20/RConn1
  Temperature Sensor20/RConn2 -- PS-Simulink Converter30/LConn1
  Temperature Sensor22/RConn2 -- PS-Simulink Converter32/LConn1
  Switch20/RConn2 -- Voltage Sensor24/RConn2 -- Voltage Sensor14/LConn1 -- R22/LConn1 -- Batt22/RConn1
  Switch16/RConn2 -- R18/LConn1 -- Batt18/RConn1 -- Voltage Sensor21/LConn1 -- Voltage Sensor20/RConn2
  Switch14/RConn2 -- R16/LConn1 -- Batt16/RConn1 -- Voltage Sensor19/LConn1 -- Voltage Sensor18/RConn2
  Switch22/RConn2 -- R24/LConn1 -- Batt24/RConn1 -- Voltage Sensor16/LConn1 -- Voltage Sensor15/RConn2
  Switch19/RConn2 -- Voltage Sensor24/LConn1 -- Voltage Sensor23/RConn2 -- Batt21/RConn1 -- R21/LConn1
  Switch21/RConn2 -- Voltage Sensor14/RConn2 -- Voltage Sensor15/LConn1 -- Batt23/RConn1 -- R23/LConn1
  Switch12/RConn2 -- R14/LConn1 -- Batt14/RConn1 -- Voltage Sensor13/RConn2 -- Voltage Sensor17/LConn1
  Switch15/RConn2 -- Voltage Sensor19/RConn2 -- Voltage Sensor20/LConn1 -- R17/LConn1 -- Batt17/RConn1
  Switch13/RConn2 -- R15/LConn1 -- Batt15/RConn1 -- Voltage Sensor18/LConn1 -- Voltage Sensor17/RConn2
  Switch17/RConn2 -- R19/LConn1 -- Batt19/RConn1 -- Voltage Sensor21/RConn2 -- Voltage Sensor22/LConn1
  Switch18/RConn2 -- Voltage Sensor22/RConn2 -- Voltage Sensor23/LConn1 -- Batt20/RConn1 -- R20/LConn1
  Switch23/RConn2 -- Batt25/RConn1 -- Voltage Sensor16/RConn2
  Switch14/RConn1 -- Simulink-PS Converter19/RConn1
  Switch22/RConn1 -- Simulink-PS Converter15/RConn1
  Voltage Sensor21/RConn1 -- PS-Simulink Converter47/LConn1
  Switch13/LConn1 -- R14/RConn1
  PS-Simulink Converter39/LConn1 -- Voltage Sensor13/RConn1
  Voltage Sensor19/RConn1 -- PS-Simulink Converter44/LConn1
  Switch21/RConn1 -- Simulink-PS Converter23/RConn1
  Voltage Sensor23/RConn1 -- PS-Simulink Converter41/LConn1
  Voltage Sensor18/RConn1 -- PS-Simulink Converter36/LConn1
  Voltage Sensor17/RConn1 -- PS-Simulink Converter45/LConn1
  Switch23/LConn1 -- R24/RConn1
  Switch12/LConn1 -- R13/RConn1
  PS-Simulink Converter38/LConn1 -- Voltage Sensor22/RConn1
  Switch18/RConn1 -- Simulink-PS Converter24/RConn1
  Switch12/RConn1 -- Simulink-PS Converter18/RConn1
  Switch13/RConn1 -- Simulink-PS Converter13/RConn1
  Switch15/LConn1 -- R16/RConn1
  Switch20/LConn1 -- R21/RConn1
  Switch14/LConn1 -- R15/RConn1
  Voltage Sensor14/RConn1 -- PS-Simulink Converter40/LConn1
  Voltage Sensor20/RConn1 -- PS-Simulink Converter46/LConn1
  Voltage Sensor16/RConn1 -- PS-Simulink Converter43/LConn1
  Switch18/LConn1 -- R19/RConn1
  Switch21/LConn1 -- R22/RConn1
  Switch17/LConn1 -- R18/RConn1
  Switch16/RConn1 -- Simulink-PS Converter20/RConn1
  Switch19/RConn1 -- Simulink-PS Converter22/RConn1
  Switch16/LConn1 -- R17/RConn1
  Voltage Sensor15/RConn1 -- PS-Simulink Converter42/LConn1
  Switch17/RConn1 -- Simulink-PS Converter21/RConn1
  Switch23/RConn1 -- Simulink-PS Converter16/RConn1
  Switch20/RConn1 -- Simulink-PS Converter14/RConn1
  Switch22/LConn1 -- R23/RConn1
  Switch19/LConn1 -- R20/RConn1
  Switch15/RConn1 -- Simulink-PS Converter17/RConn1
  Voltage Sensor24/RConn1 -- PS-Simulink Converter37/LConn1
